simulink model "Mieszanie_substancji"  (R2015a)
settings: Solver=ode45  StartTime=0.0  StopTime=1200  FixedStep=0.1  RelTol=1e-3
settings Model: Creator=Karol  LastModifiedBy=lenovo
settings OptimizationCC: ExpressionDepthLimit=2147483647
settings DebuggingCC: UnderspecifiedInitializationDetection=Classic  MergeDetectMultiDrivingBlocksExec=none  SolverPrmCheckMsg=warning  StateNameClashWarn=warning

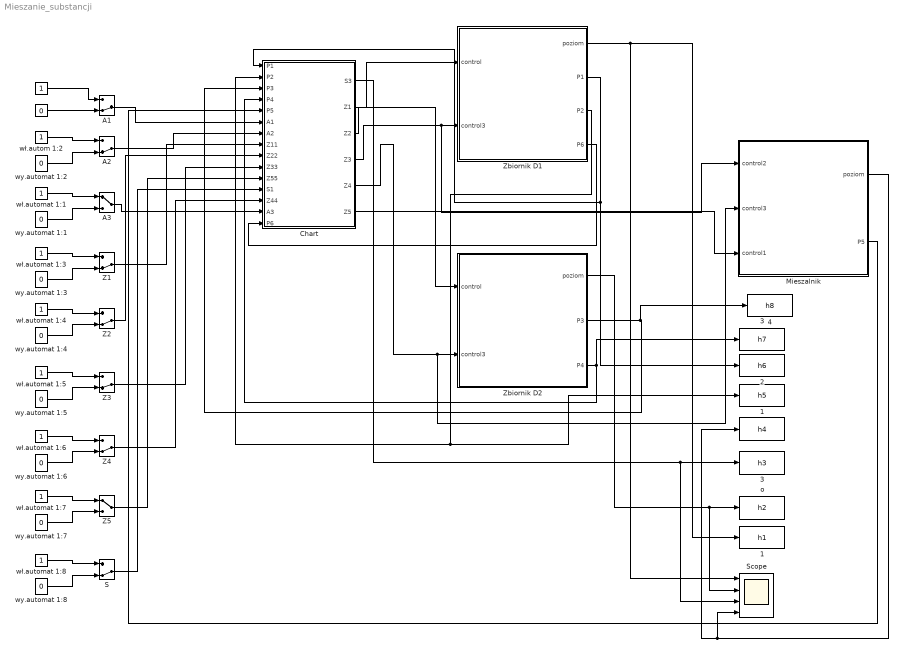
== system Mieszanie_substancji ==
  " " : Constant  Value=0
  " " : Constant
  " " : ToWorkspace  VariableName=h4  SaveFormat=Timeseries  SampleTime=-1
  " 1" : ToWorkspace  VariableName=h5  SaveFormat=Timeseries  SampleTime=-1
  " 2" : ToWorkspace  VariableName=h6  SaveFormat=Timeseries  SampleTime=-1
  " 3" : ToWorkspace  VariableName=h7  SaveFormat=Timeseries  SampleTime=-1
  " 4" : ToWorkspace  VariableName=h8  SaveFormat=Timeseries  SampleTime=-1
  1 : ToWorkspace  VariableName=h1  SaveFormat=Timeseries  SampleTime=-1
  3 : ToWorkspace  VariableName=h3  SaveFormat=Timeseries  SampleTime=-1
  A1 : ManualSwitch  CurrentSetting=0
  A2 : ManualSwitch  CurrentSetting=0
  A3 : ManualSwitch
  Chart : Stateflow chart  TreatAsAtomicUnit=on
  Mieszalnik : Subsystem
  S : ManualSwitch  CurrentSetting=0
  Scope : Scope  NumInputPorts=4
      settings: TimeRange=500  YMin=0~0~-1~0  YMax=80~80~1~300
  Z{1..4} (4 alike) : ManualSwitch  CurrentSetting=0
  Z5 : ManualSwitch
  Zbiornik D1 : Subsystem
  Zbiornik D2 : Subsystem
  "o " : ToWorkspace  VariableName=h2  SaveFormat=Timeseries  SampleTime=-1
  wy.automat 1:{1..8} (8 alike) : Constant  Value=0
  wł.autom 1:2 : Constant
  wł.automat 1:{1,3..8} (7 alike) : Constant
  wires:
  Zbiornik D1/2(P1) -> " 2"/1, Chart/1(P1)
  Zbiornik D2/3(P4) -> Chart/4(P4), " 3"/1
  Zbiornik D2/2(P3) -> " 4"/1, Chart/3(P3)
  Chart/2(Z1) -> Zbiornik D1/1(control)
  Chart/4(Z3) -> Mieszalnik/1(control2), Zbiornik D1/2(control3)
  Chart/3(Z2) -> Zbiornik D2/1(control)
  Chart/5(Z4) -> Mieszalnik/2(control3), Zbiornik D2/2(control3)
  Mieszalnik/2(P5) -> Chart/5(P5)
  Chart/6(Z5) -> Mieszalnik/3(control1)
  " "/1 -> A1/1
  " "/1 -> A1/2
  A1/1 -> Chart/6(A1)
  wł.autom 1:2/1 -> A2/1
  wy.automat 1:2/1 -> A2/2
  A2/1 -> Chart/7(A2)
  wł.automat 1:1/1 -> A3/1
  wy.automat 1:1/1 -> A3/2
  wł.automat 1:3/1 -> Z1/1
  wy.automat 1:3/1 -> Z1/2
  wł.automat 1:4/1 -> Z2/1
  wy.automat 1:4/1 -> Z2/2
  wł.automat 1:5/1 -> Z3/1
  wy.automat 1:5/1 -> Z3/2
  wł.automat 1:6/1 -> Z4/1
  wy.automat 1:6/1 -> Z4/2
  wł.automat 1:7/1 -> Z5/1
  wy.automat 1:7/1 -> Z5/2
  wł.automat 1:8/1 -> S/1
  wy.automat 1:8/1 -> S/2
  A3/1 -> Chart/14(A3)
  Z1/1 -> Chart/8(Z11)
  Z2/1 -> Chart/9(Z22)
  Z3/1 -> Chart/10(Z33)
  Z4/1 -> Chart/13(Z44)
  Z5/1 -> Chart/11(Z55)
  S/1 -> Chart/12(S1)
  Zbiornik D1/1(poziom) -> Scope/1, 1/1
  Zbiornik D1/3(P2) -> Chart/2(P2), " 1"/1
  Mieszalnik/1(poziom) -> Scope/4, " "/1
  Zbiornik D1/4(P6) -> Chart/15(P6)
  Chart/1(S3) -> Scope/3, 3/1
  Zbiornik D2/1(poziom) -> Scope/2, "o "/1

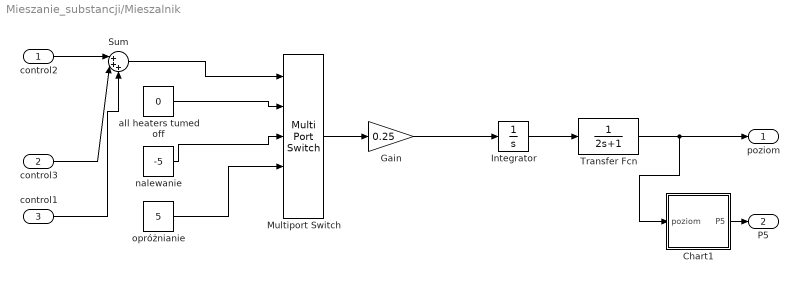
== system Mieszanie_substancji/Mieszalnik ==
  control2 : Inport
  control3 : Inport  Port=2
  control1 : Inport  Port=3
  Chart1 : Stateflow chart  TreatAsAtomicUnit=on
  Gain : Gain  Gain=0.25
  Integrator : Integrator  LimitOutput=on  UpperSaturationLimit=210.05  LowerSaturationLimit=0
  Multiport Switch : MultiPortSwitch  DataPortOrder=Zero-based contiguous  Inputs=4
  Sum : Sum  Inputs=|+++
  Transfer Fcn : TransferFcn  Denominator=[2 1]
  all heaters tumed off : Constant  Value=0
  nalewanie : Constant  Value=-5
  opróżnianie : Constant  Value=5
  poziom : Outport
  P5 : Outport  Port=2
  wires:
  Transfer Fcn/1 -> Chart1/1(poziom), poziom/1
  Chart1/1(P5) -> P5/1
  opróżnianie/1 -> Multiport Switch/4
  nalewanie/1 -> Multiport Switch/3
  all heaters tumed off/1 -> Multiport Switch/2
  Integrator/1 -> Transfer Fcn/1
  Multiport Switch/1 -> Gain/1
  Gain/1 -> Integrator/1
  control2/1 -> Sum/1
  Sum/1 -> Multiport Switch/1
  control3/1 -> Sum/2
  control1/1 -> Sum/3

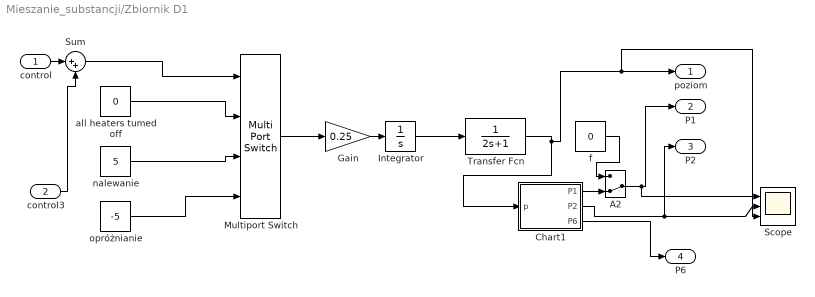
== system Mieszanie_substancji/Zbiornik D1 ==
  control : Inport
  control3 : Inport  Port=2
  A2 : ManualSwitch  CurrentSetting=0
  Chart1 : Stateflow chart  TreatAsAtomicUnit=on
  Gain : Gain  Gain=0.25
  Integrator : Integrator  LimitOutput=on  UpperSaturationLimit=101  LowerSaturationLimit=0
  Multiport Switch : MultiPortSwitch  DataPortOrder=Zero-based contiguous
  Scope : Scope  NumInputPorts=3
      settings: YMin=0~0~-5  YMax=200~2~5  SaveName=ScopeData2
  Sum : Sum  Inputs=|++
  Transfer Fcn : TransferFcn  Denominator=[2 1]
  all heaters tumed off : Constant  Value=0
  f : Constant  Value=0
  nalewanie : Constant  Value=5
  opróżnianie : Constant  Value=-5
  poziom : Outport
  P1 : Outport  Port=2
  P2 : Outport  Port=3
  P6 : Outport  Port=4
  wires:
  Chart1/2(P2) -> P2/1, Scope/2
  Transfer Fcn/1 -> Chart1/1(p), Scope/3, poziom/1
  opróżnianie/1 -> Multiport Switch/4
  nalewanie/1 -> Multiport Switch/3
  all heaters tumed off/1 -> Multiport Switch/2
  Integrator/1 -> Transfer Fcn/1
  Multiport Switch/1 -> Gain/1
  Gain/1 -> Integrator/1
  control/1 -> Sum/1
  Sum/1 -> Multiport Switch/1
  control3/1 -> Sum/2
  Chart1/3(P6) -> P6/1
  A2/1 -> Scope/1, P1/1
  Chart1/1(P1) -> A2/2
  f/1 -> A2/1

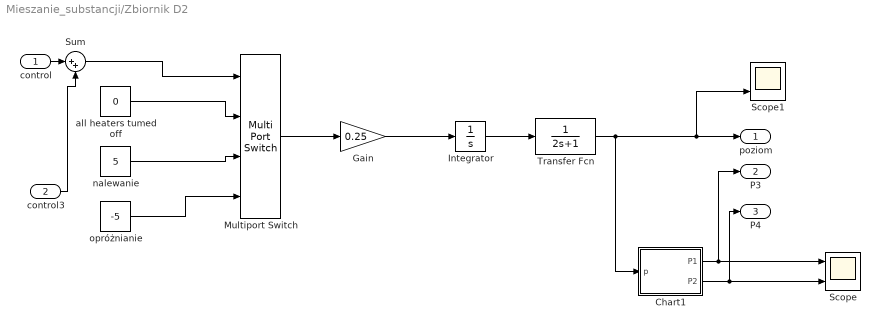
== system Mieszanie_substancji/Zbiornik D2 ==
  control : Inport
  control3 : Inport  Port=2
  Chart1 : Stateflow chart  TreatAsAtomicUnit=on
  Gain : Gain  Gain=0.25
  Integrator : Integrator  LimitOutput=on  UpperSaturationLimit=70.05  LowerSaturationLimit=0
  Multiport Switch : MultiPortSwitch  DataPortOrder=Zero-based contiguous
  Scope : Scope  NumInputPorts=2
      settings: YMin=0~0  YMax=200~1  SaveName=ScopeData4
  Scope1 : Scope  NumInputPorts=2
      settings: YMin=0~0  YMax=200~1  SaveName=ScopeData5
  Sum : Sum  Inputs=|++
  Transfer Fcn : TransferFcn  Denominator=[2 1]
  all heaters tumed off : Constant  Value=0
  nalewanie : Constant  Value=5
  opróżnianie : Constant  Value=-5
  poziom : Outport
  P3 : Outport  Port=2
  P4 : Outport  Port=3
  wires:
  opróżnianie/1 -> Multiport Switch/4
  nalewanie/1 -> Multiport Switch/3
  all heaters tumed off/1 -> Multiport Switch/2
  Integrator/1 -> Transfer Fcn/1
  Multiport Switch/1 -> Gain/1
  Transfer Fcn/1 -> Chart1/1(p), Scope1/2, poziom/1
  Gain/1 -> Integrator/1
  Chart1/1(P1) -> P3/1, Scope/1
  Chart1/2(P2) -> P4/1, Scope/2
  control/1 -> Sum/1
  Sum/1 -> Multiport Switch/1
  control3/1 -> Sum/2

== stateflow chart Mieszanie_substancji/Zbiornik D2/Chart1 ==
  state z
    entry:P2=1;
    entry:P1=0;
  state z1
    entry:P2=0;
    entry:P1=0;
  state z2
    entry:P1=1;
    entry:P2=0;
  (default) -> z
  z1 -> z2 [order 1] : [p>=70]
  z -> z1 : [p>=0.1]
  z2 -> z1 : [p<=70]
  z1 -> z [order 2] : [p<=0.1]
  data: P1 output; P2 output; p input

== stateflow chart Mieszanie_substancji/Zbiornik D1/Chart1 ==
  state z
    entry:P2=1;
    entry:P1=0;
  state z1
    entry:P2=0;
    entry:P1=0;
  state z2
    entry:P1=1;
    entry:P2=0;
  state z4
    entry:P6=1;
  (default) -> z
  z1 -> z2 [order 1] : [p>=70]
  z -> z1 : [p>=0.1]
  z2 -> z1 [order 1] : [p<=69.9]
  z1 -> z [order 2] : [p<=0.2]
  z4 -> z2 : [p>=100]
  z2 -> z4 [order 2] : [p>100]
  data: P1 output; P2 output; p input; P6 output

== stateflow chart Mieszanie_substancji/Chart ==
  state awria
    entry:S3=0;
    entry:Z1=0;
    entry:Z2=0;
    entry:Z3=0;
    entry:Z4=0;
    entry:Z5=0;
  state f2
    entry:Z2=1;
  state f1
    entry:Z1=1;
  state f3
    entry:Z3=2;
  state Manual
    entry:Z1=0;
    entry:Z2=0;
    entry:Z3=0;
    entry:Z4=0;
    entry:Z5=0;
    entry:S3=0;
  state poczatek
  state yyu
    entry:S3=0;
    entry:Z1=1;
    entry:Z2=1;
    entry:Z3=0;
    entry:Z4=0;
    entry:Z5=1;
  state ku
    entry:S3=0;
    entry:Z1=0;
    entry:Z2=1;
    entry:Z3=0;
    entry:Z4=0;
    entry:Z5=1;
  state jkuh
    entry:S3=0;
    entry:Z1=0;
    entry:Z2=0;
    entry:Z3=0;
    entry:Z4=0;
    entry:Z5=1;
  state wd
    entry:S3=0;
    entry:Z1=0;
    entry:Z2=1;
    entry:Z3=2;
    entry:Z4=0;
    entry:Z5=0;
  state automat11
    entry:S3=0;
    entry:Z1=1;
    entry:Z2=1;
    entry:Z3=0;
    entry:Z4=0;
    entry:Z5=0;
  state dwd
    entry:S3=0;
    entry:Z1=0;
    entry:Z2=0;
    entry:Z3=2;
    entry:Z4=0;
    entry:Z5=0;
  state f4
    entry:Z4=2;
  state dwg
    entry:S3=1;
    entry:Z1=0;
    entry:Z2=0;
    entry:Z3=0;
    entry:Z4=2;
    entry:Z5=0;
  state f5
    entry:Z5=1;
  state f6
    entry:S3=1;
  state dw
    entry:S3=0;
    entry:Z1=1;
    entry:Z2=0;
    entry:Z3=0;
    entry:Z4=0;
    entry:Z5=0;
  state wdw
    entry:S3=0;
    entry:Z1=0;
    entry:Z2=1;
    entry:Z3=0;
    entry:Z4=0;
    entry:Z5=0;
  state hj
    entry:S3=0;
  state wdgf
    entry:S3=1;
    entry:Z1=0;
    entry:Z2=0;
    entry:Z3=0;
    entry:Z4=0;
    entry:Z5=0;
  state we
    entry:S3=0;
    entry:Z1=0;
    entry:Z2=0;
    entry:Z3=2;
    entry:Z4=0;
    entry:Z5=0;
  state ku1
    entry:S3=0;
    entry:Z1=0;
    entry:Z2=1;
    entry:Z3=0;
    entry:Z4=0;
    entry:Z5=1;
  state yyu1
    entry:S3=0;
    entry:Z1=1;
    entry:Z2=1;
    entry:Z3=0;
    entry:Z4=0;
    entry:Z5=1;
  state automat12
    entry:S3=0;
    entry:Z1=1;
    entry:Z2=1;
    entry:Z3=0;
    entry:Z4=0;
    entry:Z5=0;
  state d3
    entry:S3=0;
    entry:Z1=1;
    entry:Z2=1;
    entry:Z3=0;
    entry:Z4=0;
    entry:Z5=0;
  state d4
    entry:S3=0;
    entry:Z1=0;
    entry:Z2=1;
    entry:Z3=2;
    entry:Z4=0;
    entry:Z5=0;
  state d5
    entry:S3=0;
    entry:Z1=0;
    entry:Z2=1;
    entry:Z3=0;
    entry:Z4=0;
    entry:Z5=0;
  state d2
    entry:S3=0;
    entry:Z1=0;
    entry:Z2=1;
    entry:Z3=2;
    entry:Z4=0;
    entry:Z5=0;
  state jkuh1
    entry:S3=0;
    entry:Z1=0;
    entry:Z2=0;
    entry:Z3=0;
    entry:Z4=0;
    entry:Z5=1;
  state ku2
    entry:S3=0;
    entry:Z1=1;
    entry:Z2=0;
    entry:Z3=0;
    entry:Z4=0;
    entry:Z5=1;
  state d12
    entry:S3=0;
    entry:Z1=0;
    entry:Z2=0;
    entry:Z3=2;
    entry:Z4=0;
    entry:Z5=0;
  state d10
    entry:S3=0;
    entry:Z1=1;
    entry:Z2=0;
    entry:Z3=0;
    entry:Z4=0;
    entry:Z5=0;
  state d8
    entry:S3=0;
    entry:Z1=0;
    entry:Z2=0;
    entry:Z3=2;
    entry:Z4=0;
    entry:Z5=0;
  state d7
    entry:S3=1;
    entry:Z1=0;
    entry:Z2=0;
    entry:Z3=0;
    entry:Z4=2;
    entry:Z5=0;
  state hj1
  state d9
    entry:S3=0;
    entry:Z1=0;
    entry:Z2=0;
    entry:Z3=2;
    entry:Z4=0;
    entry:Z5=0;
  state d6
    entry:S3=1;
    entry:Z1=0;
    entry:Z2=0;
    entry:Z3=0;
    entry:Z4=0;
    entry:Z5=0;
  state d11
    entry:S3=0;
    entry:Z1=1;
    entry:Z2=0;
    entry:Z3=0;
    entry:Z4=0;
    entry:Z5=0;
  state d13
    entry:S3=0;
    entry:Z1=0;
    entry:Z2=0;
    entry:Z3=2;
    entry:Z4=0;
    entry:Z5=0;
  yyu -> awria [order 3] : [P6==1]
  hj -> poczatek [order 2] : [A1==0]
  yyu -> automat11 [order 1] : [P5==1]
  Manual -> f2 [order 3] : [Z22==1]
  f2 -> Manual : [Z22==0]
  f1 -> Manual : [Z11==0]
  Manual -> f1 [order 2] : [Z11==1]
  dw -> awria [order 2] : [P6==1]
  automat11 -> awria [order 3] : [P6==1]
  ku -> wd [order 1] : [P5==1]
  (default) -> poczatek [order 2]
  Manual -> f3 [order 4] : [Z33==1]
  f3 -> Manual : [Z33==0]
  (default) -> Manual [order 1] : [A3==1]
  wd -> dwd [order 1] : [P3==1]
  Manual -> poczatek [order 1] : [A3==0]
  automat11 -> wd [order 1] : [P1==1&P5==1]
  Manual -> f4 [order 5] : [Z44==1]
  yyu -> ku [order 2] : [P1==1]
  ku -> jkuh [order 2] : [P3==1]
  jkuh -> dwd : [P5==1]
  poczatek -> automat11 [order 1] : [A1==1]
  f4 -> Manual : [Z44==0]
  Manual -> f5 [order 6] : [Z55==1]
  f5 -> Manual : [Z55==0]
  Manual -> f6 [order 7] : [S1==1]
  f6 -> Manual : [S1==0]
  dwd -> dwg : [P2==1]
  automat11 -> dw [order 2] : [P3==1]
  wd -> wdw [order 2] : [P2==1]
  hj1 -> poczatek [order 2] : [A1==0]
  poczatek -> automat12 [order 2] : [A2==1]
  hj -> yyu [order 1] : [A1==1]
  wdw -> dwg : [P3==1]
  wdgf -> hj : after(40,sec)
  we -> dwg : [P2==1]
  dw -> we [order 1] : [P1==1&P5==1]
  dwg -> wdgf : [P4==1]
  yyu1 -> automat12 [order 2] : [P5==1]
  ku1 -> d2 [order 2] : [P5==1]
  yyu1 -> ku1 [order 1] : [P1==1]
  ku1 -> jkuh1 [order 1] : [P3==1]
  d4 -> d5 [order 1] : [P2==1]
  d2 -> d3 [order 1] : [P2==1]
  d3 -> d4 : [P1==1]
  automat12 -> d2 [order 1] : [P1==1&P5==1]
  yyu1 -> ku2 [order 3] : [P3==1]
  ku2 -> jkuh1 [order 2] : [P1==1]
  jkuh1 -> d9 : [P5==1]
  automat12 -> d10 [order 2] : [P3==1]
  d4 -> d8 [order 2] : [P3==1]
  d5 -> d7 : [P3==1]
  hj1 -> yyu1 [order 1] : [A2==1]
  d2 -> d12 [order 2] : [P3==1]
  ku2 -> d10 [order 1] : [P5==1]
  d8 -> d7 : [P2==1]
  d13 -> d7 : [P2==1]
  d12 -> d11 : [P2==1]
  d10 -> d9 : [P1==1]
  d7 -> d6 : [P4==1]
  d6 -> hj1 : after(40,sec)
  d9 -> d11 : [P2==1]
  d11 -> d13 : [P1==1]
  data: P1 input; P2 input; P3 input; P4 input; S3 output; Z1 output; Z2 output; Z3 output; Z4 output; Z5 output; P5 input; A1 input; A2 input; Z11 input; Z22 input; Z33 input; Z55 input; S1 input; Z44 input; A3 input; P6 input

== stateflow chart Mieszanie_substancji/Mieszalnik/Chart1 ==
  state f1
    entry:P5=1;
  state f2
    entry:P5=0;
  (default) -> f1
  f1 -> f2 : [poziom>0.1]
  f2 -> f1 : [poziom<=0.1]
  data: poziom input; P5 output double
